simulink model "IEEE123bus_v2019b_Phasor_DPL"  (R2019b)
settings: Solver=VariableStepAuto  StartTime=0.0  StopTime=100  FixedStep=Ts  RelTol=1e-3
InitFcn:
  | a=1; % Loading Factor
  | Ts=0.1;% For Delay Blocks in Voltage Regulator Controls
  | 
  | % Simulation data for the IEEE 123 Node Test Feeder model
  | mi2km = 1.60934;%  miles to km conversion
  | ft2km = 0.0003048; % feet to km conversion
  | ms2F = 1*1e-6/(2*pi*60);% microsiemens to Farads conversion
  | 
  | %% Configuration 1
  | % Series Resitance and Reactance - ohm/mile
  | R_1 = [0.4576 0.1560 0.1535;0.1560 0.4666 0.1580;0.1535 0.1580 0.4615];
  | X_1 = [1.0780 0.5017 0.3849;0.5017 1.0482 0.4236;0.3849 0.4236 1.0651];
  | % charging susceptance - microsiemens/mile
  | B_1 = [5.6765 -1.8319 -0.6982;-1.8319 5.9809 -1.1645;-0.6982 -1.1645 5.3971];
  | 
  | R_1 = R_1/mi2km;
  | L_1 = (X_1/(2*pi*60))/mi2km;
  | C_1 =(B_1*ms2F)/mi2km;
  | 
  | %% Configuration 2 - series reactance - ohm/mile
  | R_2 = [0.4666 0.1580 0.1560;0.1580 0.4615 0.1535;0.1560 0.1535 0.4576];
  | X_2 = [1.0482 0.4236 0.5017;0.4236 1.0651 0.3849;0.5017 0.3849 1.0780];
  | % charging susceptance - microsiemens/mile
  | B_2 = [5.9809 -1.1645 -1.8319;-1.1645 5.3971 -0.6982;-1.8319 -0.6982 5.6765];
  | 
  | R_2 = R_2/mi2km;
  | L_2 = (X_2/(2*pi*60))/mi2km;
  | C_2 =(B_2*ms2F)/mi2km;
  | 
  | %% Configuration 3 - series reactance - ohm/mile
  | R_3 = [0.4615 0.1535 0.1580;0.1535 0.4576 0.1560;0.1580 0.1560 0.4666];
  | X_3 = [1.0651 0.3849 0.4236;0.3849 1.0780 0.5017;0.4236 0.5017 1.0482];
  | % charging susceptance - microsiemens/mile
  | B_3 = [5.3971 -0.6982 -1.1645;-0.6982 5.6765 -1.8319; -1.1645 -1.8319 5.9809];
  | 
  | R_3 = R_3/mi2km;
  | L_3 = (X_3/(2*pi*60))/mi2km;
  | C_3 =(B_3*ms2F)/mi2km;
  | 
  | %% Configuration 4 - series reactance - ohm/mile
  | R_4 = [0.4615 0.1580 0.1535;0.1580 0.4666 0.1560;0.1535 0.1560 0.4576];
  | X_4 = [1.0651 0.4236 0.3849;0.4236 1.0482 0.5017;0.3849 0.5017 1.0780];
  | % charging susceptance - microsiemens/mile
  | B_4 = [5.3971 -1.1645 -0.6982;-1.1645 5.9809 -1.8319;-0.6982 -1.8319 5.6765];
  | 
  | R_4 = R_4/mi2km;
  | L_4 = (X_4/(2*pi*60))/mi2km;
  | C_4 =(B_4*ms2F)/mi2km;
  | 
  | %% Configuration 5 - series reactance - ohm/mile
  | R_5 = [0.4666 0.1560 0.1580;0.1560 0.4576 0.1535;0.1580 0.1535 0.4615];
  | X_5 = [1.0482 0.5017 0.4236;0.5017 1.0780 0.3849;0.4236 0.3849 1.0651];
  | % charging susceptance - microsiemens/mile
  | B_5 = [5.9809 -1.8319 -1.1645;-1.8319 5.6765 -0.6982;-1.1645 -0.6982 5.3971];
  | 
  | R_5 = R_5/mi2km;
  | L_5 = (X_5/(2*pi*60))/mi2km;
  | C_5 =(B_5*ms2F)/mi2km;
  | 
  | %% Configuration 6 - series reactance - ohm/mile
  | ... (+68 lines)
undefined symbols (not defined in the file or in its folder): D1, Delta, find_system, j
libraries: powerlib x686, powerlib_meascontrol x31
(part 4 of 7)

== system IEEE123bus_v2019b_Phasor_DPL/96 ==
  2 : powerlib/Measurements/Three-Phase V-I Measurement  VoltageMeasurement=phase-to-ground  SetLabelV=on  LabelV=V96  Vpu=off  VpuLL=off  CurrentMeasurement=no  SetLabelI=on  LabelI=I800  Ipu=off  Pbase=100e6  Vbase=24900  OutputType=Complex  PhasorSimulation=on  PSBequivalent=0
      settings: SourceProductName=Simscape Electrical
  Ground82 : powerlib/Elements/Ground  LConnTagsString=a
      settings: SourceProductName=Simscape Electrical
  Ground83 : powerlib/Elements/Ground  LConnTagsString=a
      settings: SourceProductName=Simscape Electrical
  b : PMIOPort  Side=Right
  B : PMIOPort  Port=2  Side=Left
  connections:
  2/LConn2 -- B/RConn1
  2/RConn2 -- b/RConn1
  2/LConn1 -- 2/LConn3 -- Ground83/LConn1
  2/RConn1 -- 2/RConn3 -- Ground82/LConn1

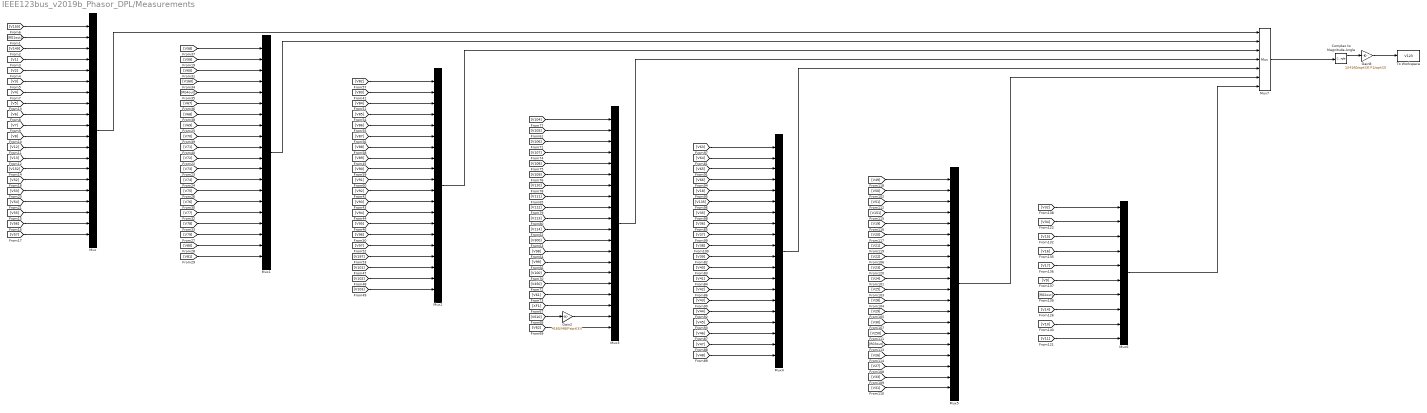
== system IEEE123bus_v2019b_Phasor_DPL/Measurements ==
  Complex to Magnitude-Angle : ComplexToMagnitudeAngle
  Gain2 : Gain  Gain=4160/(480*sqrt(3))
  Gain8 : Gain  Gain=1/(4160/sqrt(3))*1/sqrt(2)
  Mux{,1..5} (6 alike) : Mux  Inputs=20
  Mux6 : Mux  Inputs=10
  Mux7 : Mux  Inputs=7
  To Workspace : ToWorkspace  VariableName=V123  SampleTime=.1
  wires:
  Gain8/1 -> To Workspace/1
  [V150] -> Mux/1
  [RG1out] -> Mux/2
  [V149] -> Mux/3
  [V1] -> Mux/4
  [V2] -> Mux/5
  [V3] -> Mux/6
  [V4] -> Mux/7
  [V5] -> Mux/8
  [V6] -> Mux/9
  [V7] -> Mux/10
  [V8] -> Mux/11
  [V12] -> Mux/12
  [V13] -> Mux/13
  [V152] -> Mux/14
  [V52] -> Mux/15
  [V53] -> Mux/16
  [V54] -> Mux/17
  [V55] -> Mux/18
  [V56] -> Mux/19
  [V57] -> Mux/20
  [V58] -> Mux1/1
  [V59] -> Mux1/2
  [V60] -> Mux1/3
  [V160] -> Mux1/4
  [RG4out] -> Mux1/5
  [V67] -> Mux1/6
  [V68] -> Mux1/7
  [V69] -> Mux1/8
  [V70] -> Mux1/9
  [V71] -> Mux1/10
  [V72] -> Mux1/11
  [V73] -> Mux1/12
  [V74] -> Mux1/13
  [V75] -> Mux1/14
  [V76] -> Mux1/15
  [V77] -> Mux1/16
  [V78] -> Mux1/17
  [V79] -> Mux1/18
  [V80] -> Mux1/19
  [V81] -> Mux1/20
  [V82] -> Mux2/1
  [V83] -> Mux2/2
  [V84] -> Mux2/3
  [V85] -> Mux2/4
  [V86] -> Mux2/5
  [V87] -> Mux2/6
  [V88] -> Mux2/7
  [V89] -> Mux2/8
  [V90] -> Mux2/9
  [V91] -> Mux2/10
  [V92] -> Mux2/11
  [V93] -> Mux2/12
  [V94] -> Mux2/13
  [V95] -> Mux2/14
  [V96] -> Mux2/15
  [V97] -> Mux2/16
  [V197] -> Mux2/17
  [V101] -> Mux2/18
  [V102] -> Mux2/19
  [V103] -> Mux2/20
  [V104] -> Mux3/1
  [V105] -> Mux3/2
  [V106] -> Mux3/3
  [V107] -> Mux3/4
  [V108] -> Mux3/5
  [V109] -> Mux3/6
  [V110] -> Mux3/7
  [V111] -> Mux3/8
  [V112] -> Mux3/9
  [V113] -> Mux3/10
  [V114] -> Mux3/11
  [V300] -> Mux3/12
  [V98] -> Mux3/13
  [V99] -> Mux3/14
  [V100] -> Mux3/15
  [V450] -> Mux3/16
  [V61] -> Mux3/17
  [XF1] -> Mux3/18
  [V610] -> Gain2/1
  [V62] -> Mux3/20
  [V63] -> Mux4/1
  [V64] -> Mux4/2
  [V65] -> Mux4/3
  [V66] -> Mux4/4
  [V18] -> Mux4/5
  [V135] -> Mux4/6
  [V35] -> Mux4/7
  [V36] -> Mux4/8
  [V37] -> Mux4/9
  [V38] -> Mux4/10
  [V39] -> Mux4/11
  [V40] -> Mux4/12
  [V41] -> Mux4/13
  [V42] -> Mux4/14
  [V43] -> Mux4/15
  [V44] -> Mux4/16
  [V45] -> Mux4/17
  [V46] -> Mux4/18
  [V47] -> Mux4/19
  [V48] -> Mux4/20
  [V49] -> Mux5/1
  [V50] -> Mux5/2
  [V51] -> Mux5/3
  [V151] -> Mux5/4
  [V19] -> Mux5/5
  [V20] -> Mux5/6
  [V21] -> Mux5/7
  [V22] -> Mux5/8
  [V23] -> Mux5/9
  [V24] -> Mux5/10
  [V25] -> Mux5/11
  [V28] -> Mux5/12
  [V29] -> Mux5/13
  [V30] -> Mux5/14
  [V250] -> Mux5/15
  [RG3out] -> Mux5/16
  [V26] -> Mux5/17
  [V27] -> Mux5/18
  [V33] -> Mux5/19
  [V31] -> Mux5/20
  Mux1/1 -> Mux7/2
  Mux/1 -> Mux7/1
  Mux2/1 -> Mux7/3
  Mux3/1 -> Mux7/4
  Mux4/1 -> Mux7/5
  Mux5/1 -> Mux7/6
  Gain2/1 -> Mux3/19
  [V32] -> Mux6/1
  [V34] -> Mux6/2
  [V15] -> Mux6/3
  [V16] -> Mux6/4
  [V17] -> Mux6/5
  [V9] -> Mux6/6
  [RG2out] -> Mux6/7
  [V14] -> Mux6/8
  [V10] -> Mux6/9
  [V11] -> Mux6/10
  Mux6/1 -> Mux7/7
  Complex to Magnitude-Angle/1 -> Gain8/1
  Mux7/1 -> Complex to Magnitude-Angle/1

== system IEEE123bus_v2019b_Phasor_DPL/RG2in ==
  2 : powerlib/Measurements/Three-Phase V-I Measurement  VoltageMeasurement=phase-to-ground  SetLabelV=on  LabelV=RG2in  Vpu=off  VpuLL=off  CurrentMeasurement=no  SetLabelI=on  LabelI=I800  Ipu=off  Pbase=100e6  Vbase=24900  OutputType=Complex  PhasorSimulation=on  PSBequivalent=0
      settings: SourceProductName=Simscape Electrical
  Ground82 : powerlib/Elements/Ground  LConnTagsString=a
      settings: SourceProductName=Simscape Electrical
  Ground83 : powerlib/Elements/Ground  LConnTagsString=a
      settings: SourceProductName=Simscape Electrical
  a : PMIOPort  Side=Right
  A : PMIOPort  Port=2  Side=Left
  connections:
  A/RConn1 -- 2/LConn1
  a/RConn1 -- 2/RConn1
  2/LConn2 -- 2/LConn3 -- Ground83/LConn1
  2/RConn2 -- 2/RConn3 -- Ground82/LConn1

== system IEEE123bus_v2019b_Phasor_DPL/RG2out ==
  2 : powerlib/Measurements/Three-Phase V-I Measurement  VoltageMeasurement=phase-to-ground  SetLabelV=on  LabelV=RG2out  Vpu=off  VpuLL=off  CurrentMeasurement=no  SetLabelI=on  LabelI=I800  Ipu=off  Pbase=100e6  Vbase=24900  OutputType=Complex  PhasorSimulation=on  PSBequivalent=0
      settings: SourceProductName=Simscape Electrical
  Ground82 : powerlib/Elements/Ground  LConnTagsString=a
      settings: SourceProductName=Simscape Electrical
  Ground83 : powerlib/Elements/Ground  LConnTagsString=a
      settings: SourceProductName=Simscape Electrical
  a : PMIOPort  Side=Right
  A : PMIOPort  Port=2  Side=Left
  connections:
  Ground82/LConn1 -- 2/RConn3 -- 2/RConn2
  Ground83/LConn1 -- 2/LConn3 -- 2/LConn2
  a/RConn1 -- 2/RConn1
  A/RConn1 -- 2/LConn1

== system IEEE123bus_v2019b_Phasor_DPL/RG3in ==
  1 : powerlib/Measurements/Three-Phase V-I Measurement  VoltageMeasurement=phase-to-ground  SetLabelV=on  LabelV=RG3in  Vpu=off  VpuLL=off  CurrentMeasurement=yes  SetLabelI=on  LabelI=IRG3in  Ipu=off  Pbase=100e6  Vbase=24900  OutputType=Complex  PhasorSimulation=on  PSBequivalent=0
      settings: SourceProductName=Simscape Electrical
  Ground1 : powerlib/Elements/Ground  LConnTagsString=a
      settings: SourceProductName=Simscape Electrical
  Ground2 : powerlib/Elements/Ground  LConnTagsString=a
      settings: SourceProductName=Simscape Electrical
  A : PMIOPort  Side=Left
  a : PMIOPort  Port=2  Side=Right
  C : PMIOPort  Port=3  Side=Left
  c : PMIOPort  Port=4  Side=Right
  connections:
  A/RConn1 -- 1/LConn1
  a/RConn1 -- 1/RConn1
  C/RConn1 -- 1/LConn3
  1/RConn2 -- Ground1/LConn1
  c/RConn1 -- 1/RConn3
  1/LConn2 -- Ground2/LConn1

== system IEEE123bus_v2019b_Phasor_DPL/RG3out ==
  1 : powerlib/Measurements/Three-Phase V-I Measurement  VoltageMeasurement=phase-to-ground  SetLabelV=on  LabelV=RG3out  Vpu=off  VpuLL=off  CurrentMeasurement=no  SetLabelI=on  LabelI=I800  Ipu=off  Pbase=100e6  Vbase=24900  OutputType=Complex  PhasorSimulation=on  PSBequivalent=0
      settings: SourceProductName=Simscape Electrical
  Ground1 : powerlib/Elements/Ground  LConnTagsString=a
      settings: SourceProductName=Simscape Electrical
  Ground2 : powerlib/Elements/Ground  LConnTagsString=a
      settings: SourceProductName=Simscape Electrical
  A : PMIOPort  Side=Left
  a : PMIOPort  Port=2  Side=Right
  C : PMIOPort  Port=3  Side=Left
  c : PMIOPort  Port=4  Side=Right
  connections:
  1/LConn2 -- Ground2/LConn1
  c/RConn1 -- 1/RConn3
  1/RConn2 -- Ground1/LConn1
  C/RConn1 -- 1/LConn3
  a/RConn1 -- 1/RConn1
  A/RConn1 -- 1/LConn1

== system IEEE123bus_v2019b_Phasor_DPL/Regulator 1 Three Phase Ganged SVR ==
  note: Here the voltage of one phase is used to control taps of all phases
      | The phase A voltage is monitored and used to control taps of other phases
  Ganged Line Drop Compensator : Subsystem  mask{pNom=5e6/3, fNom=60, vNom=4160/sqrt(3), ptRatio=20, Comp=[3 7.5]}
      mask prompts: pNom "Nominal power (VA)"; fNom "Nominal frequency (Hz)"; vNom "Nominal voltage (Vrms)"; ptRatio "PT Ratio"; Comp "Compensator Settings [R (V) X(V)]"
      mask init:
      | Rc=Comp(1);
      | Xc=Comp(2);
  Mux : Mux  Inputs=3
  Single Phase SVR_A : Subsystem  LoadFcn=find_system(gcs,'FollowLinks', 'on', 'LookUnderMasks', 'all');  mask(Single-Phase OLTC){pNom=5e6/3, fNom=60, vNom=4160/sqrt(3), ctRatio=700, ptRatio=20, DeltaU=0.00625, TapMinMax=[-16 16], InitialTap=7, TapSelectionTime=8, RegulatorOn=on, Regulator=[120/120  2/120  2]}
      mask prompts: pNom "Nominal Power (VA)"; fNom "Nominal Frequency (Hz)"; vNom "Nominal Voltage (Vrms)"; ctRatio "Primary CT Rating (A)"; ptRatio "PT Ratio"; DeltaU "Voltage Step Per Tap (pu)"; TapMinMax "Minimum and Maximum Tap Positions"; InitialTap "Initial Tap Position"; TapSelectionTime "Tap Selection Time (s)"; RegulatorOn "Voltage Regulator"; Regulator "Voltage Regulator [ Vref(pu) DeadBand(pu)  Delay(s)]"
      mask help:
      | Models a single-phase On Load Tap Changer (OLTC). The single-phase primary of multi-tap winding is modeled with a Variable-Ratio Transformer block.
      |
      | The transformer voltage ratio U2/U1 (in pu) is given by:
      |                 U2/U1= 1/ (1+TapPosition*DeltaU)
      | Tap position 0 corresponds to nominal voltage ratio.
      |
      | When Voltage regulator is 'on',  voltage regulator asks for a tap change if:
      |                  abs(Vm-Vref)>DeadBand/2  during a time  t > Delay.
      |
      | where 'Vm' is voltage measured at regulating point and Vref is reference voltage.
      | With line drop compensation, Vm=Vsec-Isec(R+jX)
      mask init:
      | RegulatorVref=Regulator(1);
      | RegulatorDeadBand=Regulator(2);
      | RegulatorDelay=Regulator(3);
      mask TypeOptions RegulatorOn: off | on
      mask Callback RegulatorOn:
      | tempMaskVis=get_param(gcb,'MaskVisibilities');
      | if strcmp(get_param(gcb,'RegulatorOn'),'on')
      | 	tempMaskVis{11}='on';
      | 	set_param(gcb,'MaskVisibilities',tempMaskVis);
      | else
      | 	tempMaskVis{11}='off';
      | 	set_param(gcb,'MaskVisibilities',tempMaskVis);
      | end
      mask DialogControl Container8 Prompt: Setup
      mask DialogControl Container13 Prompt: Regulator Parameters
  Single Phase SVR_B : Subsystem  LoadFcn=find_system(gcs,'FollowLinks', 'on', 'LookUnderMasks', 'all');  mask(Single-Phase OLTC){pNom=5e6/3, fNom=60, vNom=4160/sqrt(3), ctRatio=700, ptRatio=20, DeltaU=0.00625, TapMinMax=[-16 16], InitialTap=7, TapSelectionTime=8, RegulatorOn=on, Regulator=[120/120  2/120  2]}
      mask prompts: pNom "Nominal Power (VA)"; fNom "Nominal Frequency (Hz)"; vNom "Nominal Voltage (Vrms)"; ctRatio "Primary CT Rating (A)"; ptRatio "PT Ratio"; DeltaU "Voltage Step Per Tap (pu)"; TapMinMax "Minimum and Maximum Tap Positions"; InitialTap "Initial Tap Position"; TapSelectionTime "Tap Selection Time (s)"; RegulatorOn "Voltage Regulator"; Regulator "Voltage Regulator [ Vref(pu) DeadBand(pu)  Delay(s)]"
      mask help:
      | Models a single-phase On Load Tap Changer (OLTC). The single-phase primary of multi-tap winding is modeled with a Variable-Ratio Transformer block.
      |
      | The transformer voltage ratio U2/U1 (in pu) is given by:
      |                 U2/U1= 1/ (1+TapPosition*DeltaU)
      | Tap position 0 corresponds to nominal voltage ratio.
      |
      | When Voltage regulator is 'on',  voltage regulator asks for a tap change if:
      |                  abs(Vm-Vref)>DeadBand/2  during a time  t > Delay.
      |
      | where 'Vm' is voltage measured at regulating point and Vref is reference voltage.
      | With line drop compensation, Vm=Vsec-Isec(R+jX)
      mask init:
      | RegulatorVref=Regulator(1);
      | RegulatorDeadBand=Regulator(2);
      | RegulatorDelay=Regulator(3);
      mask TypeOptions RegulatorOn: off | on
      mask Callback RegulatorOn:
      | tempMaskVis=get_param(gcb,'MaskVisibilities');
      | if strcmp(get_param(gcb,'RegulatorOn'),'on')
      | 	tempMaskVis{11}='on';
      | 	set_param(gcb,'MaskVisibilities',tempMaskVis);
      | else
      | 	tempMaskVis{11}='off';
      | 	set_param(gcb,'MaskVisibilities',tempMaskVis);
      | end
      mask DialogControl Container8 Prompt: Setup
      mask DialogControl Container13 Prompt: Regulator Parameters
  Single Phase SVR_C : Subsystem  LoadFcn=find_system(gcs,'FollowLinks', 'on', 'LookUnderMasks', 'all');  mask(Single-Phase OLTC){pNom=5e6/3, fNom=60, vNom=4160/sqrt(3), ctRatio=700, ptRatio=20, DeltaU=0.00625, TapMinMax=[-16 16], InitialTap=7, TapSelectionTime=8, RegulatorOn=on, Regulator=[120/120  2/120  2]}
      mask prompts: pNom "Nominal Power (VA)"; fNom "Nominal Frequency (Hz)"; vNom "Nominal Voltage (Vrms)"; ctRatio "Primary CT Rating (A)"; ptRatio "PT Ratio"; DeltaU "Voltage Step Per Tap (pu)"; TapMinMax "Minimum and Maximum Tap Positions"; InitialTap "Initial Tap Position"; TapSelectionTime "Tap Selection Time (s)"; RegulatorOn "Voltage Regulator"; Regulator "Voltage Regulator [ Vref(pu) DeadBand(pu)  Delay(s)]"
      mask help:
      | Models a single-phase On Load Tap Changer (OLTC). The single-phase primary of multi-tap winding is modeled with a Variable-Ratio Transformer block.
      |
      | The transformer voltage ratio U2/U1 (in pu) is given by:
      |                 U2/U1= 1/ (1+TapPosition*DeltaU)
      | Tap position 0 corresponds to nominal voltage ratio.
      |
      | When Voltage regulator is 'on',  voltage regulator asks for a tap change if:
      |                  abs(Vm-Vref)>DeadBand/2  during a time  t > Delay.
      |
      | where 'Vm' is voltage measured at regulating point and Vref is reference voltage.
      | With line drop compensation, Vm=Vsec-Isec(R+jX)
      mask init:
      | RegulatorVref=Regulator(1);
      | RegulatorDeadBand=Regulator(2);
      | RegulatorDelay=Regulator(3);
      mask TypeOptions RegulatorOn: off | on
      mask Callback RegulatorOn:
      | tempMaskVis=get_param(gcb,'MaskVisibilities');
      | if strcmp(get_param(gcb,'RegulatorOn'),'on')
      | 	tempMaskVis{11}='on';
      | 	set_param(gcb,'MaskVisibilities',tempMaskVis);
      | else
      | 	tempMaskVis{11}='off';
      | 	set_param(gcb,'MaskVisibilities',tempMaskVis);
      | end
      mask DialogControl Container8 Prompt: Setup
      mask DialogControl Container13 Prompt: Regulator Parameters
  A : PMIOPort  Side=Left
  a : PMIOPort  Port=2  Side=Right
  B : PMIOPort  Port=3  Side=Left
  b : PMIOPort  Port=4  Side=Right
  C : PMIOPort  Port=5  Side=Left
  c : PMIOPort  Port=6  Side=Right
  Tap : Outport
  tag scope: Vr1=global
  wires:
  [Vm] -> Single Phase SVR_C/1(Vm)
  [Vm] -> Single Phase SVR_B/1(Vm)
  [Vm] -> Single Phase SVR_A/1(Vm)
  Ganged Line Drop Compensator/1(Vm) -> [Vr1], [Vm]
  Single Phase SVR_A/3(Vsec) -> Ganged Line Drop Compensator/2(Vsec)
  Single Phase SVR_A/2(Isec) -> Ganged Line Drop Compensator/1(Isec)
  Single Phase SVR_A/1(Tap) -> Mux/1
  Single Phase SVR_B/1(Tap) -> Mux/2
  Single Phase SVR_C/1(Tap) -> Mux/3
  Mux/1 -> Tap/1
  connections:
  Single Phase SVR_A/RConn1 -- a/RConn1
  Single Phase SVR_A/LConn1 -- A/RConn1
  Single Phase SVR_B/LConn1 -- B/RConn1
  Single Phase SVR_B/RConn1 -- b/RConn1
  Single Phase SVR_C/LConn1 -- C/RConn1
  Single Phase SVR_C/RConn1 -- c/RConn1

== system IEEE123bus_v2019b_Phasor_DPL/Regulator 2 ==
  Single Phase SVR_A : Subsystem  LoadFcn=find_system(gcs,'FollowLinks', 'on', 'LookUnderMasks', 'all');  mask(Single-Phase OLTC){pNom=5e6/3, fNom=60, vNom=4160/sqrt(3), ctRatio=50, ptRatio=20, DeltaU=0.00625, TapMinMax=[-16 16], InitialTap=-1, TapSelectionTime=8, RegulatorOn=on, Regulator=[120/120  2/120  12], Comp=[0.4 0.4]}
      mask prompts: pNom "Nominal Power (VA)"; fNom "Nominal Frequency (Hz)"; vNom "Nominal Voltage (Vrms)"; ctRatio "Primary CT Rating (A)"; ptRatio "PT Ratio"; DeltaU "Voltage Step Per Tap (pu)"; TapMinMax "Minimum and Maximum Tap Positions"; InitialTap "Initial Tap Position"; TapSelectionTime "Tap Selection Time (s)"; RegulatorOn "Voltage Regulator"; Regulator "Voltage Regulator [ Vref(pu) DeadBand(pu)  Delay(s)]"; Comp "Compensator Settings [R (V) X(V)]"
      mask help:
      | Models a single-phase On Load Tap Changer (OLTC). The single-phase primary of multi-tap winding is modeled with a Variable-Ratio Transformer block.
      |
      | The transformer voltage ratio U2/U1 (in pu) is given by:
      |                 U2/U1= 1/ (1+TapPosition*DeltaU)
      | Tap position 0 corresponds to nominal voltage ratio.
      |
      | When Voltage regulator is 'on',  voltage regulator asks for a tap change if:
      |                  abs(Vm-Vref)>DeadBand/2  during a time  t > Delay.
      |
      | where 'Vm' is voltage measured at regulating point and Vref is reference voltage.
      | With line drop compensation, Vm=Vsec-Isec(R+jX)
      mask init:
      | RegulatorVref=Regulator(1);
      | RegulatorDeadBand=Regulator(2);
      | RegulatorDelay=Regulator(3);
      | Rc=Comp(1);
      | Xc=Comp(2);
      mask TypeOptions RegulatorOn: off | on
      mask Callback RegulatorOn:
      | tempMaskVis=get_param(gcb,'MaskVisibilities');
      | if strcmp(get_param(gcb,'RegulatorOn'),'on')
      | 	tempMaskVis{11}='on';
      | 	set_param(gcb,'MaskVisibilities',tempMaskVis);
      | else
      | 	tempMaskVis{11}='off';
      | 	set_param(gcb,'MaskVisibilities',tempMaskVis);
      | end
      | if strcmp(get_param(gcb,'RegulatorOn'),'on')
      | 	tempMaskVis{12}='on';
      | 	set_param(gcb,'MaskVisibilities',tempMaskVis);
      | else
      | 	tempMaskVis{12}='off';
      | 	set_param(gcb,'MaskVisibilities',tempMaskVis);
      | end
      mask DialogControl Container8 Prompt: Setup
      mask DialogControl Container13 Prompt: Regulator Parameters
  A : PMIOPort  Side=Left
  a : PMIOPort  Port=2  Side=Right
  Tap : Outport
  wires:
  Single Phase SVR_A/1(Tap) -> Tap/1
  connections:
  Single Phase SVR_A/RConn1 -- a/RConn1
  Single Phase SVR_A/LConn1 -- A/RConn1

== system IEEE123bus_v2019b_Phasor_DPL/Regulator 3 ==
  Mux : Mux  Inputs=2
  Single Phase SVR_A : Subsystem  LoadFcn=find_system(gcs,'FollowLinks', 'on', 'LookUnderMasks', 'all');  mask(Single-Phase OLTC){pNom=5e6/3, fNom=60, vNom=4160/sqrt(3), ctRatio=50, ptRatio=20, DeltaU=0.00625, TapMinMax=[-16 16], InitialTap=0, TapSelectionTime=8, RegulatorOn=on, Regulator=[120/120  1/120  12], Comp=[0.4 0.4]}
      mask prompts: pNom "Nominal Power (VA)"; fNom "Nominal Frequency (Hz)"; vNom "Nominal Voltage (Vrms)"; ctRatio "Primary CT Rating (A)"; ptRatio "PT Ratio"; DeltaU "Voltage Step Per Tap (pu)"; TapMinMax "Minimum and Maximum Tap Positions"; InitialTap "Initial Tap Position"; TapSelectionTime "Tap Selection Time (s)"; RegulatorOn "Voltage Regulator"; Regulator "Voltage Regulator [ Vref(pu) DeadBand(pu)  Delay(s)]"; Comp "Compensator Settings [R (V) X(V)]"
      mask help:
      | Models a single-phase On Load Tap Changer (OLTC). The single-phase primary of multi-tap winding is modeled with a Variable-Ratio Transformer block.
      |
      | The transformer voltage ratio U2/U1 (in pu) is given by:
      |                 U2/U1= 1/ (1+TapPosition*DeltaU)
      | Tap position 0 corresponds to nominal voltage ratio.
      |
      | When Voltage regulator is 'on',  voltage regulator asks for a tap change if:
      |                  abs(Vm-Vref)>DeadBand/2  during a time  t > Delay.
      |
      | where 'Vm' is voltage measured at regulating point and Vref is reference voltage.
      | With line drop compensation, Vm=Vsec-Isec(R+jX)
      mask init:
      | RegulatorVref=Regulator(1);
      | RegulatorDeadBand=Regulator(2);
      | RegulatorDelay=Regulator(3);
      | Rc=Comp(1);
      | Xc=Comp(2);
      mask TypeOptions RegulatorOn: off | on
      mask Callback RegulatorOn:
      | tempMaskVis=get_param(gcb,'MaskVisibilities');
      | if strcmp(get_param(gcb,'RegulatorOn'),'on')
      | 	tempMaskVis{11}='on';
      | 	set_param(gcb,'MaskVisibilities',tempMaskVis);
      | else
      | 	tempMaskVis{11}='off';
      | 	set_param(gcb,'MaskVisibilities',tempMaskVis);
      | end
      | if strcmp(get_param(gcb,'RegulatorOn'),'on')
      | 	tempMaskVis{12}='on';
      | 	set_param(gcb,'MaskVisibilities',tempMaskVis);
      | else
      | 	tempMaskVis{12}='off';
      | 	set_param(gcb,'MaskVisibilities',tempMaskVis);
      | end
      mask DialogControl Container8 Prompt: Setup
      mask DialogControl Container13 Prompt: Regulator Parameters
  Single Phase SVR_C : Subsystem  LoadFcn=find_system(gcs,'FollowLinks', 'on', 'LookUnderMasks', 'all');  mask(Single-Phase OLTC){pNom=5e6/3, fNom=60, vNom=4160/sqrt(3), ctRatio=50, ptRatio=20, DeltaU=0.00625, TapMinMax=[-16 16], InitialTap=-1, TapSelectionTime=8, RegulatorOn=on, Regulator=[120/120  1/120  12], Comp=[0.4 0.4]}
      mask prompts: pNom "Nominal Power (VA)"; fNom "Nominal Frequency (Hz)"; vNom "Nominal Voltage (Vrms)"; ctRatio "Primary CT Rating (A)"; ptRatio "PT Ratio"; DeltaU "Voltage Step Per Tap (pu)"; TapMinMax "Minimum and Maximum Tap Positions"; InitialTap "Initial Tap Position"; TapSelectionTime "Tap Selection Time (s)"; RegulatorOn "Voltage Regulator"; Regulator "Voltage Regulator [ Vref(pu) DeadBand(pu)  Delay(s)]"; Comp "Compensator Settings [R (V) X(V)]"
      mask help:
      | Models a single-phase On Load Tap Changer (OLTC). The single-phase primary of multi-tap winding is modeled with a Variable-Ratio Transformer block.
      |
      | The transformer voltage ratio U2/U1 (in pu) is given by:
      |                 U2/U1= 1/ (1+TapPosition*DeltaU)
      | Tap position 0 corresponds to nominal voltage ratio.
      |
      | When Voltage regulator is 'on',  voltage regulator asks for a tap change if:
      |                  abs(Vm-Vref)>DeadBand/2  during a time  t > Delay.
      |
      | where 'Vm' is voltage measured at regulating point and Vref is reference voltage.
      | With line drop compensation, Vm=Vsec-Isec(R+jX)
      mask init:
      | RegulatorVref=Regulator(1);
      | RegulatorDeadBand=Regulator(2);
      | RegulatorDelay=Regulator(3);
      | Rc=Comp(1);
      | Xc=Comp(2);
      mask TypeOptions RegulatorOn: off | on
      mask Callback RegulatorOn:
      | tempMaskVis=get_param(gcb,'MaskVisibilities');
      | if strcmp(get_param(gcb,'RegulatorOn'),'on')
      | 	tempMaskVis{11}='on';
      | 	set_param(gcb,'MaskVisibilities',tempMaskVis);
      | else
      | 	tempMaskVis{11}='off';
      | 	set_param(gcb,'MaskVisibilities',tempMaskVis);
      | end
      | if strcmp(get_param(gcb,'RegulatorOn'),'on')
      | 	tempMaskVis{12}='on';
      | 	set_param(gcb,'MaskVisibilities',tempMaskVis);
      | else
      | 	tempMaskVis{12}='off';
      | 	set_param(gcb,'MaskVisibilities',tempMaskVis);
      | end
      mask DialogControl Container8 Prompt: Setup
      mask DialogControl Container13 Prompt: Regulator Parameters
  A : PMIOPort  Side=Left
  a : PMIOPort  Port=2  Side=Right
  C : PMIOPort  Port=3  Side=Left
  c : PMIOPort  Port=4  Side=Right
  Taps : Outport
  wires:
  Single Phase SVR_A/1(Tap) -> Mux/1
  Single Phase SVR_C/1(Tap) -> Mux/2
  Mux/1 -> Taps/1
  connections:
  Single Phase SVR_A/LConn1 -- A/RConn1
  Single Phase SVR_C/LConn1 -- C/RConn1
  Single Phase SVR_A/RConn1 -- a/RConn1
  Single Phase SVR_C/RConn1 -- c/RConn1

== system IEEE123bus_v2019b_Phasor_DPL/Regulator 4 ==
  Mux : Mux  Inputs=3
  Single Phase SVR_A : Subsystem  LoadFcn=find_system(gcs,'FollowLinks', 'on', 'LookUnderMasks', 'all');  mask(Single-Phase OLTC){pNom=5e6/3, fNom=60, vNom=4160/sqrt(3), ctRatio=300, ptRatio=20, DeltaU=0.00625, TapMinMax=[-16 16], InitialTap=8, TapSelectionTime=8, RegulatorOn=on, Regulator=[124/120  2/120  12], Comp=[0.6 1.3]}
      mask prompts: pNom "Nominal Power (VA)"; fNom "Nominal Frequency (Hz)"; vNom "Nominal Voltage (Vrms)"; ctRatio "Primary CT Rating (A)"; ptRatio "PT Ratio"; DeltaU "Voltage Step Per Tap (pu)"; TapMinMax "Minimum and Maximum Tap Positions"; InitialTap "Initial Tap Position"; TapSelectionTime "Tap Selection Time (s)"; RegulatorOn "Voltage Regulator"; Regulator "Voltage Regulator [ Vref(pu) DeadBand(pu)  Delay(s)]"; Comp "Compensator Settings [R (V) X(V)]"
      mask help:
      | Models a single-phase On Load Tap Changer (OLTC). The single-phase primary of multi-tap winding is modeled with a Variable-Ratio Transformer block.
      |
      | The transformer voltage ratio U2/U1 (in pu) is given by:
      |                 U2/U1= 1/ (1+TapPosition*DeltaU)
      | Tap position 0 corresponds to nominal voltage ratio.
      |
      | When Voltage regulator is 'on',  voltage regulator asks for a tap change if:
      |                  abs(Vm-Vref)>DeadBand/2  during a time  t > Delay.
      |
      | where 'Vm' is voltage measured at regulating point and Vref is reference voltage.
      | With line drop compensation, Vm=Vsec-Isec(R+jX)
      mask init:
      | RegulatorVref=Regulator(1);
      | RegulatorDeadBand=Regulator(2);
      | RegulatorDelay=Regulator(3);
      | Rc=Comp(1);
      | Xc=Comp(2);
      mask TypeOptions RegulatorOn: off | on
      mask Callback RegulatorOn:
      | tempMaskVis=get_param(gcb,'MaskVisibilities');
      | if strcmp(get_param(gcb,'RegulatorOn'),'on')
      | 	tempMaskVis{11}='on';
      | 	set_param(gcb,'MaskVisibilities',tempMaskVis);
      | else
      | 	tempMaskVis{11}='off';
      | 	set_param(gcb,'MaskVisibilities',tempMaskVis);
      | end
      | if strcmp(get_param(gcb,'RegulatorOn'),'on')
      | 	tempMaskVis{12}='on';
      | 	set_param(gcb,'MaskVisibilities',tempMaskVis);
      | else
      | 	tempMaskVis{12}='off';
      | 	set_param(gcb,'MaskVisibilities',tempMaskVis);
      | end
      mask DialogControl Container8 Prompt: Setup
      mask DialogControl Container13 Prompt: Regulator Parameters
  Single Phase SVR_B : Subsystem  LoadFcn=find_system(gcs,'FollowLinks', 'on', 'LookUnderMasks', 'all');  mask(Single-Phase OLTC){pNom=5e6/3, fNom=60, vNom=4160/sqrt(3), ctRatio=300, ptRatio=20, DeltaU=0.00625, TapMinMax=[-16 16], InitialTap=1, TapSelectionTime=8, RegulatorOn=on, Regulator=[124/120  2/120  12], Comp=[0.6 1.3]}
      mask prompts: pNom "Nominal Power (VA)"; fNom "Nominal Frequency (Hz)"; vNom "Nominal Voltage (Vrms)"; ctRatio "Primary CT Rating (A)"; ptRatio "PT Ratio"; DeltaU "Voltage Step Per Tap (pu)"; TapMinMax "Minimum and Maximum Tap Positions"; InitialTap "Initial Tap Position"; TapSelectionTime "Tap Selection Time (s)"; RegulatorOn "Voltage Regulator"; Regulator "Voltage Regulator [ Vref(pu) DeadBand(pu)  Delay(s)]"; Comp "Compensator Settings [R (V) X(V)]"
      mask help:
      | Models a single-phase On Load Tap Changer (OLTC). The single-phase primary of multi-tap winding is modeled with a Variable-Ratio Transformer block.
      |
      | The transformer voltage ratio U2/U1 (in pu) is given by:
      |                 U2/U1= 1/ (1+TapPosition*DeltaU)
      | Tap position 0 corresponds to nominal voltage ratio.
      |
      | When Voltage regulator is 'on',  voltage regulator asks for a tap change if:
      |                  abs(Vm-Vref)>DeadBand/2  during a time  t > Delay.
      |
      | where 'Vm' is voltage measured at regulating point and Vref is reference voltage.
      | With line drop compensation, Vm=Vsec-Isec(R+jX)
      mask init:
      | RegulatorVref=Regulator(1);
      | RegulatorDeadBand=Regulator(2);
      | RegulatorDelay=Regulator(3);
      | Rc=Comp(1);
      | Xc=Comp(2);
      mask TypeOptions RegulatorOn: off | on
      mask Callback RegulatorOn:
      | tempMaskVis=get_param(gcb,'MaskVisibilities');
      | if strcmp(get_param(gcb,'RegulatorOn'),'on')
      | 	tempMaskVis{11}='on';
      | 	set_param(gcb,'MaskVisibilities',tempMaskVis);
      | else
      | 	tempMaskVis{11}='off';
      | 	set_param(gcb,'MaskVisibilities',tempMaskVis);
      | end
      | if strcmp(get_param(gcb,'RegulatorOn'),'on')
      | 	tempMaskVis{12}='on';
      | 	set_param(gcb,'MaskVisibilities',tempMaskVis);
      | else
      | 	tempMaskVis{12}='off';
      | 	set_param(gcb,'MaskVisibilities',tempMaskVis);
      | end
      mask DialogControl Container8 Prompt: Setup
      mask DialogControl Container13 Prompt: Regulator Parameters
  Single Phase SVR_C : Subsystem  LoadFcn=find_system(gcs,'FollowLinks', 'on', 'LookUnderMasks', 'all');  mask(Single-Phase OLTC){pNom=5e6/3, fNom=60, vNom=4160/sqrt(3), ctRatio=300, ptRatio=20, DeltaU=0.00625, TapMinMax=[-16 16], InitialTap=5, TapSelectionTime=8, RegulatorOn=on, Regulator=[124/120  2/120  12], Comp=[0.6 1.3]}
      mask prompts: pNom "Nominal Power (VA)"; fNom "Nominal Frequency (Hz)"; vNom "Nominal Voltage (Vrms)"; ctRatio "Primary CT Rating (A)"; ptRatio "PT Ratio"; DeltaU "Voltage Step Per Tap (pu)"; TapMinMax "Minimum and Maximum Tap Positions"; InitialTap "Initial Tap Position"; TapSelectionTime "Tap Selection Time (s)"; RegulatorOn "Voltage Regulator"; Regulator "Voltage Regulator [ Vref(pu) DeadBand(pu)  Delay(s)]"; Comp "Compensator Settings [R (V) X(V)]"
      mask help:
      | Models a single-phase On Load Tap Changer (OLTC). The single-phase primary of multi-tap winding is modeled with a Variable-Ratio Transformer block.
      |
      | The transformer voltage ratio U2/U1 (in pu) is given by:
      |                 U2/U1= 1/ (1+TapPosition*DeltaU)
      | Tap position 0 corresponds to nominal voltage ratio.
      |
      | When Voltage regulator is 'on',  voltage regulator asks for a tap change if:
      |                  abs(Vm-Vref)>DeadBand/2  during a time  t > Delay.
      |
      | where 'Vm' is voltage measured at regulating point and Vref is reference voltage.
      | With line drop compensation, Vm=Vsec-Isec(R+jX)
      mask init:
      | RegulatorVref=Regulator(1);
      | RegulatorDeadBand=Regulator(2);
      | RegulatorDelay=Regulator(3);
      | Rc=Comp(1);
      | Xc=Comp(2);
      mask TypeOptions RegulatorOn: off | on
      mask Callback RegulatorOn:
      | tempMaskVis=get_param(gcb,'MaskVisibilities');
      | if strcmp(get_param(gcb,'RegulatorOn'),'on')
      | 	tempMaskVis{11}='on';
      | 	set_param(gcb,'MaskVisibilities',tempMaskVis);
      | else
      | 	tempMaskVis{11}='off';
      | 	set_param(gcb,'MaskVisibilities',tempMaskVis);
      | end
      | if strcmp(get_param(gcb,'RegulatorOn'),'on')
      | 	tempMaskVis{12}='on';
      | 	set_param(gcb,'MaskVisibilities',tempMaskVis);
      | else
      | 	tempMaskVis{12}='off';
      | 	set_param(gcb,'MaskVisibilities',tempMaskVis);
      | end
      mask DialogControl Container8 Prompt: Setup
      mask DialogControl Container13 Prompt: Regulator Parameters
  A : PMIOPort  Side=Left
  a : PMIOPort  Port=2  Side=Right
  B : PMIOPort  Port=3  Side=Left
  b : PMIOPort  Port=4  Side=Right
  C : PMIOPort  Port=5  Side=Left
  c : PMIOPort  Port=6  Side=Right
  Tap : Outport
  wires:
  Mux/1 -> Tap/1
  Single Phase SVR_C/1(Tap) -> Mux/3
  Single Phase SVR_B/1(Tap) -> Mux/2
  Single Phase SVR_A/1(Tap) -> Mux/1
  connections:
  Single Phase SVR_C/RConn1 -- c/RConn1
  Single Phase SVR_C/LConn1 -- C/RConn1
  Single Phase SVR_B/RConn1 -- b/RConn1
  Single Phase SVR_B/LConn1 -- B/RConn1
  Single Phase SVR_A/LConn1 -- A/RConn1
  Single Phase SVR_A/RConn1 -- a/RConn1

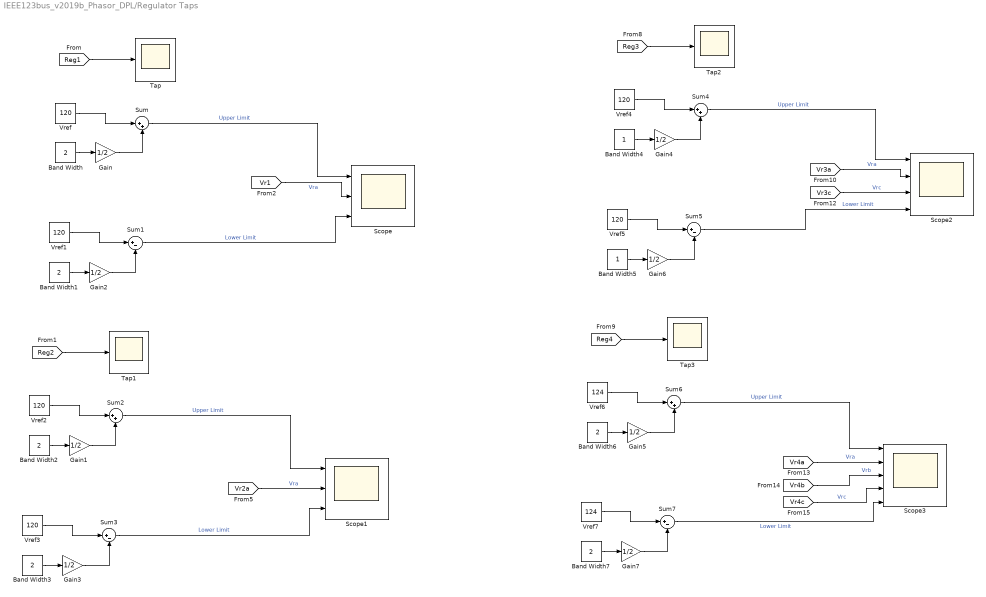
== system IEEE123bus_v2019b_Phasor_DPL/Regulator Taps ==
  Band Width{,1..3,6..7} (6 alike) : Constant  Value=2
  Band Width4 : Constant
  Band Width5 : Constant
  Gain{,1..7} (8 alike) : Gain  Gain=1/2
  Scope : Scope  NumInputPorts=3
  Scope1 : Scope  NumInputPorts=3
  Scope2 : Scope  NumInputPorts=4
  Scope3 : Scope  NumInputPorts=5
  Sum{,2,4,6} (4 alike) : Sum  Inputs=|++
  Sum{1,3,5,7} (4 alike) : Sum  Inputs=|+-
  Tap{,1..3} (4 alike) : Scope
  Vref{,1..5} (6 alike) : Constant  Value=120
  Vref6 : Constant  Value=124
  Vref7 : Constant  Value=124
  wires:
  Vref/1 -> Sum/1
  Gain2/1 -> Sum1/2
  Band Width/1 -> Gain/1
  Gain/1 -> Sum/2
  [Reg1] -> Tap/1
  Band Width1/1 -> Gain2/1
  Sum/1 -> Scope/1  "Upper Limit"
  Vref1/1 -> Sum1/1
  Sum1/1 -> Scope/3  "Lower Limit"
  [Vr1] -> Scope/2  "Vra"
  [Vr2a] -> Scope1/2  "Vra"
  Sum3/1 -> Scope1/3  "Lower Limit"
  Vref3/1 -> Sum3/1
  Sum2/1 -> Scope1/1  "Upper Limit"
  Band Width3/1 -> Gain3/1
  [Reg2] -> Tap1/1
  Gain1/1 -> Sum2/2
  Band Width2/1 -> Gain1/1
  Gain3/1 -> Sum3/2
  Vref2/1 -> Sum2/1
  Vref6/1 -> Sum6/1
  Gain7/1 -> Sum7/2
  Band Width6/1 -> Gain5/1
  Gain5/1 -> Sum6/2
  [Reg4] -> Tap3/1
  [Vr4c] -> Scope3/4  "Vrc"
  Band Width7/1 -> Gain7/1
  Sum6/1 -> Scope3/1  "Upper Limit"
  Vref7/1 -> Sum7/1
  Sum7/1 -> Scope3/5  "Lower Limit"
  [Vr4b] -> Scope3/3  "Vrb"
  [Vr4a] -> Scope3/2  "Vra"
  [Vr3a] -> Scope2/2  "Vra"
  Sum5/1 -> Scope2/4  "Lower Limit"
  Vref5/1 -> Sum5/1
  Sum4/1 -> Scope2/1  "Upper Limit"
  Band Width5/1 -> Gain6/1
  [Vr3c] -> Scope2/3  "Vrc"
  [Reg3] -> Tap2/1
  Gain4/1 -> Sum4/2
  Band Width4/1 -> Gain4/1
  Gain6/1 -> Sum5/2
  Vref4/1 -> Sum4/1

== system IEEE123bus_v2019b_Phasor_DPL/Substation Power ==
  note: TOTAL
  note: From Benchmark Document
      |
      | SYSTEM PHASE PHASE PHASE TOTAL
      | INPUT -------(A)-------|-------(B)-------|-------(C)-------|------------------
      | kW : 1463.861 | 963.484 | 1193.153 | 3620.498
      | kVAr : 582.101 | 343.687 | 398.976 | 1324.765
  note: PHASE A
  note: PHASE B
  note: PHASE C
  Demux : Demux  Outputs=3
  Demux1 : Demux  Outputs=3
  Display{,1..7} (8 alike) : Display
  Gain{,1..7} (8 alike) : Gain  Gain=1e-3
  "Power (3ph, Phasor)" : powerlib_meascontrol/Measurements/Power (3ph, Phasor)
      settings: SourceProductName=Simscape Electrical  SourceProductBaseCode=PS
  Power (Phasor) : powerlib_meascontrol/Measurements/Power (Phasor)
      settings: SourceProductName=Simscape Electrical  SourceProductBaseCode=PS
  Power (Phasor)1 : powerlib_meascontrol/Measurements/Power (Phasor)
      settings: SourceProductName=Simscape Electrical  SourceProductBaseCode=PS
  Power (Phasor)2 : powerlib_meascontrol/Measurements/Power (Phasor)
      settings: SourceProductName=Simscape Electrical  SourceProductBaseCode=PS
  wires:
  [I150] -> "Power (3ph, Phasor)"/2
  [V150] -> "Power (3ph, Phasor)"/1
  "Power (3ph, Phasor)"/1 -> Gain/1
  "Power (3ph, Phasor)"/2 -> Gain1/1
  [V150] -> Demux/1
  [I150] -> Demux1/1
  Demux/1 -> Power (Phasor)/1
  Demux1/1 -> Power (Phasor)/2
  Demux/2 -> Power (Phasor)1/1
  Demux1/2 -> Power (Phasor)1/2
  Demux/3 -> Power (Phasor)2/1
  Demux1/3 -> Power (Phasor)2/2
  Power (Phasor)/1 -> Gain2/1
  Power (Phasor)/2 -> Gain3/1
  Power (Phasor)1/1 -> Gain4/1
  Power (Phasor)1/2 -> Gain5/1
  Power (Phasor)2/1 -> Gain6/1
  Power (Phasor)2/2 -> Gain7/1
  Gain/1 -> Display/1
  Gain1/1 -> Display1/1
  Gain2/1 -> Display2/1
  Gain3/1 -> Display3/1
  Gain4/1 -> Display4/1
  Gain5/1 -> Display5/1
  Gain6/1 -> Display6/1
  Gain7/1 -> Display7/1

== system IEEE123bus_v2019b_Phasor_DPL/Regulator 1 Three Phase Ganged SVR/Ganged Line Drop Compensator ==
  note: Vm=Vsec-Isec(Rc+jXc)
  Isec : Inport
  Vsec : Inport  Port=2
  Abs1 : Abs
  Gain4 : Gain  Gain=1/sqrt(2)
  Gain5 : Gain  Gain=Rc+j*Xc
  Gain6 : Gain  Gain=1/sqrt(2)
  Sum1 : Sum  Inputs=|+-
  Vm : Outport
  wires:
  Abs1/1 -> Vm/1
  Gain5/1 -> Sum1/2
  Isec/1 -> Gain4/1
  Gain4/1 -> Gain5/1
  Gain6/1 -> Sum1/1
  Sum1/1 -> Abs1/1
  Vsec/1 -> Gain6/1

== system IEEE123bus_v2019b_Phasor_DPL/Regulator 1 Three Phase Ganged SVR/Single Phase SVR_A ==
  Vm : Inport
  Transformer with Taps : Subsystem
  Voltage Regulator Control : Subsystem
  S : PMIOPort  Tag=PMCPort  Side=Left
  L : PMIOPort  Tag=PMCPort  Port=2  Side=Right
  Tap : Outport  VectorParamsAs1DForOutWhenUnconnected=off
  Isec : Outport  Port=2  VectorParamsAs1DForOutWhenUnconnected=off
  Vsec : Outport  Port=3  VectorParamsAs1DForOutWhenUnconnected=off
  wires:
  Transformer with Taps/2(Vsec) -> Vsec/1
  Transformer with Taps/1(Isec) -> Isec/1
  Voltage Regulator Control/1(Tap) -> Transformer with Taps/1(tap), Tap/1
  Vm/1 -> Voltage Regulator Control/1(Vm)
  connections:
  Transformer with Taps/LConn1 -- S/RConn1
  Transformer with Taps/RConn1 -- L/RConn1

== system IEEE123bus_v2019b_Phasor_DPL/Regulator 1 Three Phase Ganged SVR/Single Phase SVR_B ==
  Vm : Inport
  Transformer with Taps : Subsystem
  Voltage Regulator Control : Subsystem
  S : PMIOPort  Tag=PMCPort  Side=Left
  L : PMIOPort  Tag=PMCPort  Port=2  Side=Right
  Tap : Outport  VectorParamsAs1DForOutWhenUnconnected=off
  Isec : Outport  Port=2  VectorParamsAs1DForOutWhenUnconnected=off
  Vsec : Outport  Port=3  VectorParamsAs1DForOutWhenUnconnected=off
  wires:
  Vm/1 -> Voltage Regulator Control/1(Vm)
  Voltage Regulator Control/1(Tap) -> Transformer with Taps/1(tap), Tap/1
  Transformer with Taps/1(Isec) -> Isec/1
  Transformer with Taps/2(Vsec) -> Vsec/1
  connections:
  Transformer with Taps/RConn1 -- L/RConn1
  Transformer with Taps/LConn1 -- S/RConn1

== system IEEE123bus_v2019b_Phasor_DPL/Regulator 1 Three Phase Ganged SVR/Single Phase SVR_C ==
  Vm : Inport
  Transformer with Taps : Subsystem
  Voltage Regulator Control : Subsystem
  S : PMIOPort  Tag=PMCPort  Side=Left
  L : PMIOPort  Tag=PMCPort  Port=2  Side=Right
  Tap : Outport  VectorParamsAs1DForOutWhenUnconnected=off
  Isec : Outport  Port=2  VectorParamsAs1DForOutWhenUnconnected=off
  Vsec : Outport  Port=3  VectorParamsAs1DForOutWhenUnconnected=off
  wires:
  Transformer with Taps/2(Vsec) -> Vsec/1
  Transformer with Taps/1(Isec) -> Isec/1
  Voltage Regulator Control/1(Tap) -> Transformer with Taps/1(tap), Tap/1
  Vm/1 -> Voltage Regulator Control/1(Vm)
  connections:
  Transformer with Taps/LConn1 -- S/RConn1
  Transformer with Taps/RConn1 -- L/RConn1

== system IEEE123bus_v2019b_Phasor_DPL/Regulator 2/Single Phase SVR_A ==
  Line Drop Compensator : Subsystem
  Transformer with Taps : Subsystem
  Voltage Regulator Control : Subsystem
  S : PMIOPort  Tag=PMCPort  Side=Left
  L : PMIOPort  Tag=PMCPort  Port=2  Side=Right
  Tap : Outport  VectorParamsAs1DForOutWhenUnconnected=off
  tag scope: Vr2a=global
  wires:
  Line Drop Compensator/1(Vm) -> Voltage Regulator Control/1(Vm), [Vr2a]
  Voltage Regulator Control/1(Tap) -> Transformer with Taps/1(tap), Tap/1
  Transformer with Taps/1(Isec) -> Line Drop Compensator/1(Isec)
  Transformer with Taps/2(Vsec) -> Line Drop Compensator/2(Vsec)
  connections:
  Transformer with Taps/RConn1 -- L/RConn1
  Transformer with Taps/LConn1 -- S/RConn1

== system IEEE123bus_v2019b_Phasor_DPL/Regulator 3/Single Phase SVR_A ==
  Line Drop Compensator : Subsystem
  Transformer with Taps : Subsystem
  Voltage Regulator Control : Subsystem
  S : PMIOPort  Tag=PMCPort  Side=Left
  L : PMIOPort  Tag=PMCPort  Port=2  Side=Right
  Tap : Outport  VectorParamsAs1DForOutWhenUnconnected=off
  tag scope: Vr3a=global
  wires:
  Line Drop Compensator/1(Vm) -> Voltage Regulator Control/1(Vm), [Vr3a]
  Voltage Regulator Control/1(Tap) -> Transformer with Taps/1(tap), Tap/1
  Transformer with Taps/1(Isec) -> Line Drop Compensator/1(Isec)
  Transformer with Taps/2(Vsec) -> Line Drop Compensator/2(Vsec)
  connections:
  Transformer with Taps/RConn1 -- L/RConn1
  Transformer with Taps/LConn1 -- S/RConn1

== system IEEE123bus_v2019b_Phasor_DPL/Regulator 3/Single Phase SVR_C ==
  Line Drop Compensator : Subsystem
  Transformer with Taps : Subsystem
  Voltage Regulator Control : Subsystem
  S : PMIOPort  Tag=PMCPort  Side=Left
  L : PMIOPort  Tag=PMCPort  Port=2  Side=Right
  Tap : Outport  VectorParamsAs1DForOutWhenUnconnected=off
  tag scope: Vr3c=global
  wires:
  Transformer with Taps/2(Vsec) -> Line Drop Compensator/2(Vsec)
  Transformer with Taps/1(Isec) -> Line Drop Compensator/1(Isec)
  Voltage Regulator Control/1(Tap) -> Transformer with Taps/1(tap), Tap/1
  Line Drop Compensator/1(Vm) -> Voltage Regulator Control/1(Vm), [Vr3c]
  connections:
  Transformer with Taps/LConn1 -- S/RConn1
  Transformer with Taps/RConn1 -- L/RConn1

== system IEEE123bus_v2019b_Phasor_DPL/Regulator 4/Single Phase SVR_A ==
  Line Drop Compensator : Subsystem
  Transformer with Taps : Subsystem
  Voltage Regulator Control : Subsystem
  S : PMIOPort  Tag=PMCPort  Side=Left
  L : PMIOPort  Tag=PMCPort  Port=2  Side=Right
  Tap : Outport  VectorParamsAs1DForOutWhenUnconnected=off
  tag scope: Vr4a=global
  wires:
  Line Drop Compensator/1(Vm) -> Voltage Regulator Control/1(Vm), [Vr4a]
  Voltage Regulator Control/1(Tap) -> Tap/1, Transformer with Taps/1(tap)
  Transformer with Taps/1(Isec) -> Line Drop Compensator/1(Isec)
  Transformer with Taps/2(Vsec) -> Line Drop Compensator/2(Vsec)
  connections:
  Transformer with Taps/RConn1 -- L/RConn1
  Transformer with Taps/LConn1 -- S/RConn1

== system IEEE123bus_v2019b_Phasor_DPL/Regulator 4/Single Phase SVR_B ==
  Line Drop Compensator : Subsystem
  Transformer with Taps : Subsystem
  Voltage Regulator Control : Subsystem
  S : PMIOPort  Tag=PMCPort  Side=Left
  L : PMIOPort  Tag=PMCPort  Port=2  Side=Right
  Tap : Outport  VectorParamsAs1DForOutWhenUnconnected=off
  tag scope: Vr4b=global
  wires:
  Transformer with Taps/2(Vsec) -> Line Drop Compensator/2(Vsec)
  Transformer with Taps/1(Isec) -> Line Drop Compensator/1(Isec)
  Voltage Regulator Control/1(Tap) -> Transformer with Taps/1(tap), Tap/1
  Line Drop Compensator/1(Vm) -> Voltage Regulator Control/1(Vm), [Vr4b]
  connections:
  Transformer with Taps/LConn1 -- S/RConn1
  Transformer with Taps/RConn1 -- L/RConn1

== system IEEE123bus_v2019b_Phasor_DPL/Regulator 4/Single Phase SVR_C ==
  Line Drop Compensator : Subsystem
  Transformer with Taps : Subsystem
  Voltage Regulator Control : Subsystem
  S : PMIOPort  Tag=PMCPort  Side=Left
  L : PMIOPort  Tag=PMCPort  Port=2  Side=Right
  Tap : Outport  VectorParamsAs1DForOutWhenUnconnected=off
  tag scope: Vr4c=global
  wires:
  Line Drop Compensator/1(Vm) -> Voltage Regulator Control/1(Vm), [Vr4c]
  Voltage Regulator Control/1(Tap) -> Transformer with Taps/1(tap), Tap/1
  Transformer with Taps/1(Isec) -> Line Drop Compensator/1(Isec)
  Transformer with Taps/2(Vsec) -> Line Drop Compensator/2(Vsec)
  connections:
  Transformer with Taps/RConn1 -- L/RConn1
  Transformer with Taps/LConn1 -- S/RConn1

== system IEEE123bus_v2019b_Phasor_DPL/Regulator 1 Three Phase Ganged SVR/Single Phase SVR_A/Transformer with Taps ==
  note: Isec on CT Ratio base
  note: Vsec on Pt Ratio base
  tap : Inport
  "    " : Gain  Gain=(1/ptRatio)
  " 1" : Gain  Gain=(1/ctRatio)
  CT : powerlib/Measurements/Current Measurement  PhasorSimulation=on  OutputType=Complex  PSBequivalent=0
      settings: SourceProductName=Simscape Electrical
  Ground1 : powerlib/Elements/Ground  LConnTagsString=a
      settings: SourceProductName=Simscape Electrical
  Ground2 : powerlib/Elements/Ground  LConnTagsString=a
      settings: SourceProductName=Simscape Electrical
  Ground3 : powerlib/Elements/Ground  LConnTagsString=a
      settings: SourceProductName=Simscape Electrical
  Memory : Memory
  Memory1 : Memory
  PT : powerlib/Measurements/Voltage Measurement  PhasorSimulation=on  OutputType=Complex  PSBequivalent=0
      settings: SourceProductName=Simscape Electrical
  Tap Changing Transformer : Subsystem  mask(Tap Changing Transformer){}
      mask help: Implements a Tap changing two-winding ideal transformer with taps at secondary.
      mask Display:
      | A=[-85 -45 -44 -34 -26 -21 -20 -22 -28 -37 -47 -57 -63 -63 -54 -44 -34 -26 -21 -20 -22 -28 -37 -47 -57 -63 -63 -54 -44 -34 -26 -21 -20 -22 -28 -37 -47 -57 -63 -63 -54 -44 -34 -26 -21 -20 -22 -28 -37 -45 -45 -85];
      | B=[-50 -50 -50 -49 -45 -39 -33 -26 -21 -18 -17 -19 -22 -22 -26 -27 -25 -22 -16 -9 -3 2 6 6 4 1 1 -3 -4 -2 2 7 14 20 26 29 30 28 24 24 21 20 21 25 31 37 44 49 50 50 50 50];
      | C=[85 45 44 34 26 21 20 22 28 37 47 57 63 75 63 54 44 34 26 21 20 22 28 37 47 57 63 75 63 54 44 34 26 21 20 22 28 37 47 57 63 75 63 54 44 34 26 21 20 22 28 37 45 45 85];
      | D=[-50 -50 -50 -49 -45 -39 -33 -26 -21 -18 -17 -19 -22 -22 -22 -26 -27 -25 -22 -16 -9 -3 2 6 6 4 1 1 1 -3 -4 -2 2 7 14 20 26 29 30 28 24 24 24 21 20 21 25 31 37 44 49 50 50 50 50];
      | plot(-85,-100,85,100,A,B,C,D);
      | text(-50,-70, '1');text(40,-70, '2');
      | color('green')
      | port_label('Lconn',1,'+');port_label('Rconn',1,'+');
      | color('blue')
      | disp('N')
  L : PMIOPort  Tag=PMCPort  Side=Right
  S : PMIOPort  Port=2  Side=Left
  Isec : Outport
  Vsec : Outport  Port=2
  wires:
  tap/1 -> Tap Changing Transformer/1(Tap)
  Memory/1 -> Isec/1
  Memory1/1 -> Vsec/1
  " 1"/1 -> Memory/1
  CT/1 -> " 1"/1
  PT/1 -> "    "/1
  "    "/1 -> Memory1/1
  connections:
  Tap Changing Transformer/LConn2 -- Ground3/LConn1
  Tap Changing Transformer/LConn1 -- S/RConn1
  Tap Changing Transformer/RConn2 -- Ground2/LConn1
  CT/RConn1 -- L/RConn1
  PT/LConn1 -- CT/LConn1 -- Tap Changing Transformer/RConn1
  PT/LConn2 -- Ground1/LConn1

== system IEEE123bus_v2019b_Phasor_DPL/Regulator 1 Three Phase Ganged SVR/Single Phase SVR_A/Voltage Regulator Control ==
  Vm : Inport
  Constant : Constant  Value=RegulatorOn
  Tap Changer Control : Subsystem  mask(Tap Changer Control){MinMaxTap=TapMinMax, InitialPosition=InitialTap, MecDelay=TapSelectionTime}
      mask prompts: MinMaxTap "Minimum and maximum tap number [ Min  Max ] :"; InitialPosition "Initial tap position"; MecDelay "Mechanical delay time"
      mask init:
      | if MecDelay<=0,
      | 	MecDelay=1/60;
      | end
  Voltage regulator : Subsystem  mask{Vref=RegulatorVref*120, DeadBand=RegulatorDeadBand*120, TimeDelay=RegulatorDelay}
      mask prompts: Vref "Vref (on 120v base)"; DeadBand "Deadband (on 120v base)"; TimeDelay "Time delay (s)"
  Tap : Outport
  wires:
  Vm/1 -> Voltage regulator/1(Vmes (pu))
  Constant/1 -> Voltage regulator/3(RegOn)
  Tap Changer Control/2(Ready) -> Voltage regulator/2(Ready)
  Voltage regulator/1(Up) -> Tap Changer Control/1("Up ")
  Tap Changer Control/1(TapNo) -> Tap/1  "Tap"
  Voltage regulator/2(Down) -> Tap Changer Control/2("Down ")

== system IEEE123bus_v2019b_Phasor_DPL/Regulator 1 Three Phase Ganged SVR/Single Phase SVR_B/Transformer with Taps ==
  note: Isec on CT Ratio base
  note: Vsec on Pt Ratio base
  tap : Inport
  "    " : Gain  Gain=(1/ptRatio)
  " 1" : Gain  Gain=(1/ctRatio)
  CT : powerlib/Measurements/Current Measurement  PhasorSimulation=on  OutputType=Complex  PSBequivalent=0
      settings: SourceProductName=Simscape Electrical
  Ground1 : powerlib/Elements/Ground  LConnTagsString=a
      settings: SourceProductName=Simscape Electrical
  Ground2 : powerlib/Elements/Ground  LConnTagsString=a
      settings: SourceProductName=Simscape Electrical
  Ground3 : powerlib/Elements/Ground  LConnTagsString=a
      settings: SourceProductName=Simscape Electrical
  Memory : Memory
  Memory1 : Memory
  PT : powerlib/Measurements/Voltage Measurement  PhasorSimulation=on  OutputType=Complex  PSBequivalent=0
      settings: SourceProductName=Simscape Electrical
  Tap Changing Transformer : Subsystem  mask(Tap Changing Transformer){}
      mask help: Implements a Tap changing two-winding ideal transformer with taps at secondary.
      mask Display:
      | A=[-85 -45 -44 -34 -26 -21 -20 -22 -28 -37 -47 -57 -63 -63 -54 -44 -34 -26 -21 -20 -22 -28 -37 -47 -57 -63 -63 -54 -44 -34 -26 -21 -20 -22 -28 -37 -47 -57 -63 -63 -54 -44 -34 -26 -21 -20 -22 -28 -37 -45 -45 -85];
      | B=[-50 -50 -50 -49 -45 -39 -33 -26 -21 -18 -17 -19 -22 -22 -26 -27 -25 -22 -16 -9 -3 2 6 6 4 1 1 -3 -4 -2 2 7 14 20 26 29 30 28 24 24 21 20 21 25 31 37 44 49 50 50 50 50];
      | C=[85 45 44 34 26 21 20 22 28 37 47 57 63 75 63 54 44 34 26 21 20 22 28 37 47 57 63 75 63 54 44 34 26 21 20 22 28 37 47 57 63 75 63 54 44 34 26 21 20 22 28 37 45 45 85];
      | D=[-50 -50 -50 -49 -45 -39 -33 -26 -21 -18 -17 -19 -22 -22 -22 -26 -27 -25 -22 -16 -9 -3 2 6 6 4 1 1 1 -3 -4 -2 2 7 14 20 26 29 30 28 24 24 24 21 20 21 25 31 37 44 49 50 50 50 50];
      | plot(-85,-100,85,100,A,B,C,D);
      | text(-50,-70, '1');text(40,-70, '2');
      | color('green')
      | port_label('Lconn',1,'+');port_label('Rconn',1,'+');
      | color('blue')
      | disp('N')
  L : PMIOPort  Tag=PMCPort  Side=Right
  S : PMIOPort  Port=2  Side=Left
  Isec : Outport
  Vsec : Outport  Port=2
  wires:
  tap/1 -> Tap Changing Transformer/1(Tap)
  Memory/1 -> Isec/1
  Memory1/1 -> Vsec/1
  " 1"/1 -> Memory/1
  CT/1 -> " 1"/1
  PT/1 -> "    "/1
  "    "/1 -> Memory1/1
  connections:
  Tap Changing Transformer/LConn2 -- Ground3/LConn1
  Tap Changing Transformer/LConn1 -- S/RConn1
  Tap Changing Transformer/RConn2 -- Ground2/LConn1
  CT/RConn1 -- L/RConn1
  PT/LConn1 -- CT/LConn1 -- Tap Changing Transformer/RConn1
  PT/LConn2 -- Ground1/LConn1
